simulink subsystem "CartBase2023a"  (R2023a)
settings: Solver=VariableStepAuto  StartTime=0.0  StopTime=10.0  RelTol=1e-3
undefined symbols (not defined in the file): b, g, l, M, m
settings Model: Creator=sturton  LastModifiedBy=MY PC
settings RTWCC: GPUComputeCapability=5.0

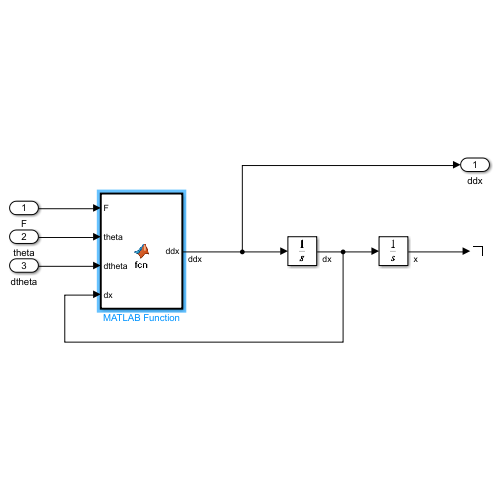
[thumbnail: Simulink's stored preview of the top-level diagram]
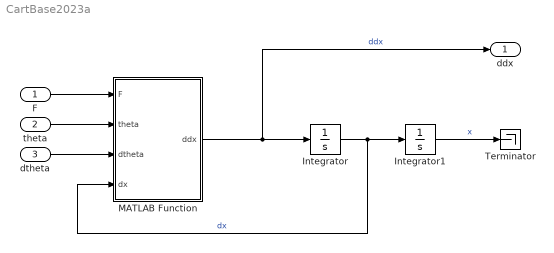
== system CartBase2023a ==
  F : Inport
  theta : Inport  Port=2
  dtheta : Inport  Port=3
  Integrator : Integrator
  Integrator1 : Integrator
  MATLAB Function : MATLAB Function  TreatAsAtomicUnit=on
  Terminator : Terminator
  ddx : Outport
  wires:
  Integrator/1 -> MATLAB Function/4(dx), Integrator1/1  "dx"
  MATLAB Function/1(ddx) -> Integrator/1, ddx/1  "ddx"
  Integrator1/1 -> Terminator/1  "x"
  theta/1 -> MATLAB Function/2(theta)
  dtheta/1 -> MATLAB Function/3(dtheta)
  F/1 -> MATLAB Function/1(F)

== matlab function CartBase2023a/MATLAB Function ==
  data: F input; theta input; dtheta input; dx input; ddx output; g parameter; M parameter; l parameter; m parameter; b parameter
function ddx = fcn(F,theta,dtheta,dx,g, M, l, m, b)

ddx = 1/(M + m*(sin(theta))^2)*(F + m*l*dtheta^2*sin(theta) -b*dx +m*g*cos(theta)*sin(theta));
end
